simulink model "LinearHidraulicDynamics"  (R2017a)
settings: Solver=VariableStepAuto  StartTime=0.0  StopTime=1  RelTol=1e-3
libraries: fl_lib x10, nesl_utility x6
settings Model: Creator=erich  LastModifiedBy=erich

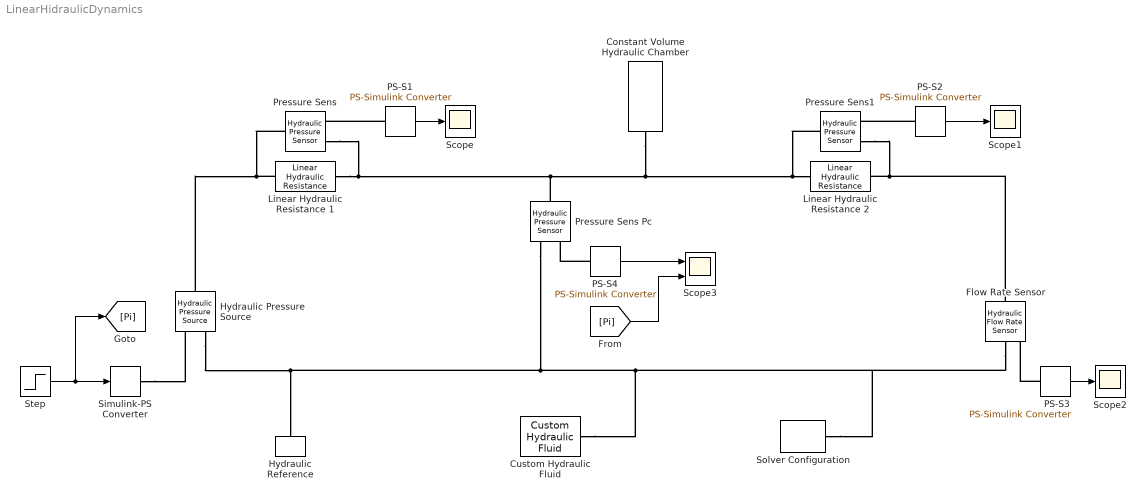
== system LinearHidraulicDynamics ==
  Constant Volume Hydraulic Chamber : fl_lib/Hydraulic/Hydraulic Elements/Constant Volume Hydraulic Chamber  ch_sp=2  wall_type=1  ch_volume=1e-4 m^3  d_in=4 m  length=5 m  pr_r_coef=1.2e-12 m/Pa  time_const=0.01 s  k_sh=1.4  pressure_specify=off  pressure_priority=High  pressure=0 psi  pressure_nominal_specify=off  pressure_nominal_unit=Pa  pressure_nominal_value=1  diameter_incr_specify=off  diameter_incr_priority=High  diameter_incr=0 m  diameter_incr_nominal_specify=off  diameter_incr_nominal_unit=m  diameter_incr_nominal_value=1  flow_rate_specify=off  flow_rate_priority=None  flow_rate=0.001 m^3/s  flow_rate_nominal_specify=off  flow_rate_nominal_unit=m^3/s  flow_rate_nominal_value=1
      settings: SourceProductName=Simscape  SourceProductBaseCode=SS
  Custom Hydraulic Fluid : fl_lib/Hydraulic/Hydraulic Utilities/Custom Hydraulic Fluid  density=1 kg/m^3  viscosity_kin=0.7978 m^2/s  bulk=2.15e9 Pa  alpha=0  range_error=2
      settings: SourceProductName=Simscape  SourceProductBaseCode=SS
  Flow Rate Sensor : fl_lib/Hydraulic/Hydraulic Sensors/Hydraulic Flow Rate Sensor
      settings: SourceProductName=Simscape
  Hydraulic Pressure Source : fl_lib/Hydraulic/Hydraulic Sources/Hydraulic Pressure Source
      settings: SourceProductName=Simscape  SourceProductBaseCode=SS
  Hydraulic Reference : fl_lib/Hydraulic/Hydraulic Elements/Hydraulic Reference
      settings: SourceProductName=Simscape
  Linear Hydraulic Resistance 1 : fl_lib/Hydraulic/Hydraulic Elements/Linear Hydraulic Resistance  resistance=2e6 Pa/(m^3/s)  q_specify=off  q_priority=None  q=0.001 m^3/s  q_nominal_specify=off  q_nominal_unit=m^3/s  q_nominal_value=1  p_specify=off  p_priority=None  p=0 Pa  p_nominal_specify=off  p_nominal_unit=Pa  p_nominal_value=1
      settings: SourceProductName=Simscape  SourceProductBaseCode=SS
  Linear Hydraulic Resistance 2 : fl_lib/Hydraulic/Hydraulic Elements/Linear Hydraulic Resistance  resistance=1e6 Pa/(m^3/s)  q_specify=off  q_priority=None  q=0.001 m^3/s  q_nominal_specify=off  q_nominal_unit=m^3/s  q_nominal_value=1  p_specify=off  p_priority=None  p=0 Pa  p_nominal_specify=off  p_nominal_unit=Pa  p_nominal_value=1
      settings: SourceProductName=Simscape  SourceProductBaseCode=SS
  PS-S{1..4} (4 alike) : nesl_utility/PS-Simulink Converter  PhysicalDomain=network_engine_domain  SubClassName=ps_output  LeftPortType=input  RightPortType=output  PseudoPeriodic=off  Frequencies=[]  Unit=1  AffineConversion=off
  Pressure Sens : fl_lib/Hydraulic/Hydraulic Sensors/Hydraulic Pressure Sensor
      settings: SourceProductName=Simscape
  Pressure Sens Pc : fl_lib/Hydraulic/Hydraulic Sensors/Hydraulic Pressure Sensor
      settings: SourceProductName=Simscape
  Pressure Sens1 : fl_lib/Hydraulic/Hydraulic Sensors/Hydraulic Pressure Sensor
      settings: SourceProductName=Simscape
  Scope : Scope
  Scope1 : Scope
  Scope2 : Scope
  Scope3 : Scope  NumInputPorts=2
  Simulink-PS Converter : nesl_utility/Simulink-PS Converter  PhysicalDomain=network_engine_domain  SubClassName=ps_input  LeftPortType=input  RightPortType=output  PseudoPeriodic=off  Frequencies=[]  NoiseDistribution=none  NoiseParameters=[]  Unit=1  AffineConversion=off  FilteringAndDerivatives=provide  SimscapeFilterOrder=1  InputFilterTimeConstant=0.001  UdotUserProvided=0
  Solver Configuration : nesl_utility/Solver Configuration  PhysicalDomain=network_engine_domain  SubClassName=solver  LeftPortType=input  RightPortType=generic  Accelerate=off  Tones=[]  Harmonics=[]  SimulateNoise=off  Profile=off  UseLocalSampling=off  EnableSwitchedLinearOptims=on  FrequencyDomain=off  UseCCode=off  RelTol=0.001  AbsTol=1e-06  MinStep=1e-09  ToWorkspace=off  RevertToSquareIcSolve=off  NumHomotopyIterations=100  PhasorMode=off  PhasorModeNumHarmonics=1  OverrideAbsTol=off  DoDC=off  ResidualTolerance=1e-09  UseLocalSolver=off  LocalSolverChoice=NE_BACKWARD_EULER_ADVANCER  LocalSolverSampleTime=0.001  DoFixedCost=off  MaxNonlinIter=3  MaxModeIter=2  LinearAlgebra=Sparse  DelaysMemoryBudget=1024  AutomaticFiltering=on  FilteringTimeConstant=0.001
  Step : Step  Time=.2  After=10  SampleTime=0
  wires:
  PS-S3/1 -> Scope2/1
  PS-S2/1 -> Scope1/1
  PS-S1/1 -> Scope/1
  Step/1 -> Simulink-PS Converter/1, [Pi]
  PS-S4/1 -> Scope3/1
  [Pi] -> Scope3/2
  connections:
  Custom Hydraulic Fluid/RConn1 -- Solver Configuration/RConn1 -- Flow Rate Sensor/RConn2 -- Pressure Sens Pc/RConn1 -- Hydraulic Pressure Source/RConn2 -- Hydraulic Reference/LConn1
  Linear Hydraulic Resistance 1/LConn1 -- Hydraulic Pressure Source/LConn1 -- Pressure Sens/LConn1
  Linear Hydraulic Resistance 1/RConn1 -- Pressure Sens/RConn1 -- Pressure Sens Pc/LConn1 -- Constant Volume Hydraulic Chamber/LConn1 -- Pressure Sens1/LConn1 -- Linear Hydraulic Resistance 2/LConn1
  Flow Rate Sensor/LConn1 -- Pressure Sens1/RConn1 -- Linear Hydraulic Resistance 2/RConn1
  PS-S3/LConn1 -- Flow Rate Sensor/RConn1
  PS-S2/LConn1 -- Pressure Sens1/RConn2
  PS-S1/LConn1 -- Pressure Sens/RConn2
  Simulink-PS Converter/RConn1 -- Hydraulic Pressure Source/RConn1
  PS-S4/LConn1 -- Pressure Sens Pc/RConn2
